simulink model "ADC"  (R2023a)
settings: Solver=FixedStepDiscrete  StartTime=0.0  StopTime=10.0  FixedStep=0.001  RelTol=1e-3
settings Model: Creator=Ilya_Andriyanov  LastModifiedBy=Ilya_Andriyanov

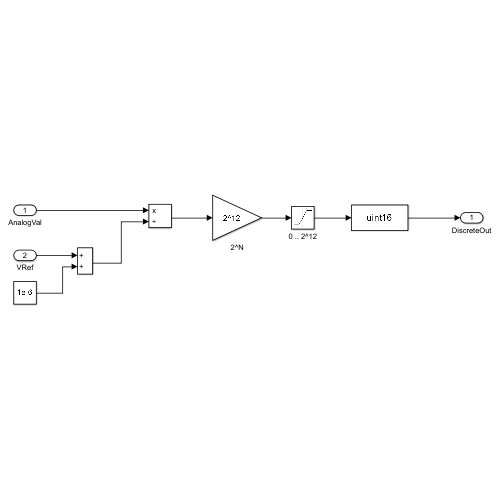
[thumbnail: Simulink's stored preview of the top-level diagram]
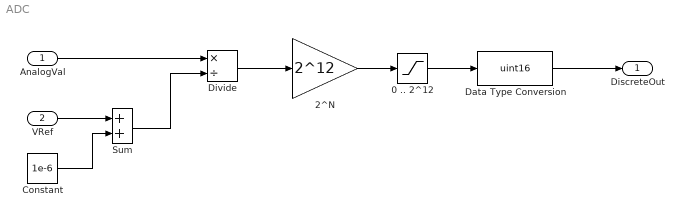
== system ADC ==
  AnalogVal : Inport
  VRef : Inport  Port=2
  0 .. 2^12 : Saturate  UpperLimit=2^12  LowerLimit=0
  2^N : Gain  Gain=2^12
  Constant : Constant  Value=1e-6
  Data Type Conversion : DataTypeConversion  OutDataTypeStr=uint16  SaturateOnIntegerOverflow=off  RndMeth=Floor
  Divide : Product  Inputs=*/
  Sum : Sum
  DiscreteOut : Outport
  wires:
  VRef/1 -> Sum/1
  Constant/1 -> Sum/2
  Sum/1 -> Divide/2
  Divide/1 -> 2^N/1
  2^N/1 -> 0 .. 2^12/1
  Data Type Conversion/1 -> DiscreteOut/1
  0 .. 2^12/1 -> Data Type Conversion/1
  AnalogVal/1 -> Divide/1
